simulink model "modello_discretizzato"  (R2021b)
settings: Solver=VariableStepAuto  StartTime=0.0  StopTime=50  RelTol=1e-3
values from neighbouring files (symbols this model uses):
  r = 1    [script.m]
  Tc = 0.20    (= 0.2)    [script.m]
undefined symbols (not defined in the file or in its folder): denom, numer
libraries: cstblocks x5
settings Model: Creator=antony  LastModifiedBy=antony

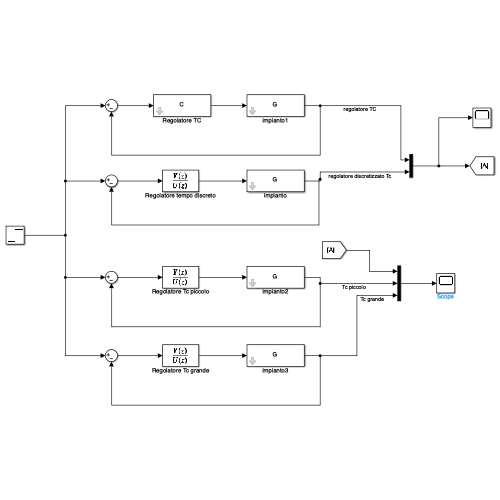
[thumbnail: Simulink's stored preview of the top-level diagram]
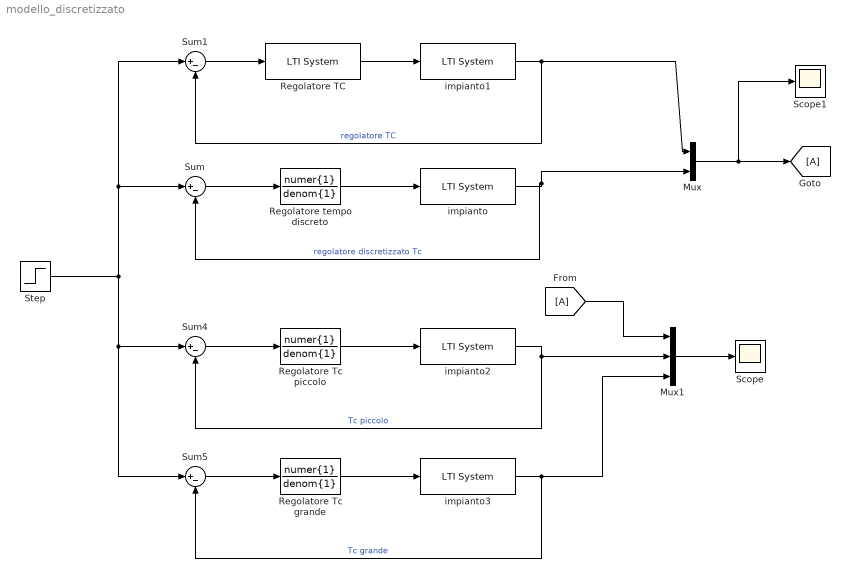
== system modello_discretizzato ==
  Mux : Mux  Inputs=2
  Mux1 : Mux  Inputs=3
  Regolatore TC : cstblocks/LTI System  sys=C  IC=[]
  Regolatore Tc grande : DiscreteTransferFcn  Numerator=numer{1}  Denominator=denom{1}  SampleTime=0.99  NumCoefDataTypeStr=int64
  Regolatore Tc piccolo : DiscreteTransferFcn  Numerator=numer{1}  Denominator=denom{1}  SampleTime=0.1  NumCoefDataTypeStr=int64
  Regolatore tempo discreto : DiscreteTransferFcn  Numerator=numer{1}  Denominator=denom{1}  SampleTime=Tc  NumCoefDataTypeStr=int64
  Scope : Scope
  Scope1 : Scope
  Step : Step  Time=0  After=r  SampleTime=0
  Sum{,1,4..5} (4 alike) : Sum  Inputs=|+-
  impianto{,1..3} (4 alike) : cstblocks/LTI System  sys=G  IC=[]
  wires:
  Step/1 -> Sum4/1, Sum5/1, Sum1/1, Sum/1
  Sum/1 -> Regolatore tempo discreto/1
  Regolatore tempo discreto/1 -> impianto/1
  impianto/1 -> Sum/2, Mux/2  "regolatore discretizzato Tc"
  Sum1/1 -> Regolatore TC/1
  impianto1/1 -> Sum1/2, Mux/1  "regolatore TC"
  Regolatore TC/1 -> impianto1/1
  Mux/1 -> Scope1/1, [A]
  Regolatore Tc piccolo/1 -> impianto2/1
  impianto2/1 -> Sum4/2, Mux1/2  "Tc piccolo"
  Sum4/1 -> Regolatore Tc piccolo/1
  Regolatore Tc grande/1 -> impianto3/1
  Sum5/1 -> Regolatore Tc grande/1
  impianto3/1 -> Mux1/3, Sum5/2  "Tc grande"
  [A] -> Mux1/1
  Mux1/1 -> Scope/1
